simulink model "dynamicANN"  (R2019b)
settings: Solver=VariableStepAuto  StartTime=0.0  StopTime=3  RelTol=1e-3
values from neighbouring files (symbols this model uses):
  a = 87.548e-3    (= 0.087548)    [main.m]
  b = 132.452e-3    (= 0.132452)    [main.m]
  d = 22.452e-3    (= 0.022452)    [main.m]
  delta = 4e-6    (= 4e-06)    [main.m]
  F1 = mass*g-F2    (= 23.4474357109)    [main.m]
  F2 = a*mass*g/(a+b)    (= 15.4982642891)    [main.m]
  g = 9.81    [main.m]
  h0 = 75e-6    (= 7.5e-05)    [main.m]
  Jd = 0.047331604    [main.m]
  Jp = 0.00075    [main.m]
  Kps = (Vmax-Vmin)/(Hmax-Hmin)    (= 1666.66666667)    [main.m]
  Ksv = 30    [main.m]
  mass = 3.970    (= 3.97)    [main.m]
  mm = F2/g    (= 1.57984345455)    [main.m]
  omega = n_rpm*2*pi/60    (= 293.215314335)    [main.m]
  s = 30e-3    (= 0.03)    [main.m]
  tau = 0.12    [main.m]
  taus = 0.00125    [main.m]
  Ts = 1/fs    (= 0.001)    [main.m]
libraries: neural x480, simulink x2
(part 1 of 11)
settings Model: Creator=Alexander  LastModifiedBy=Alexander

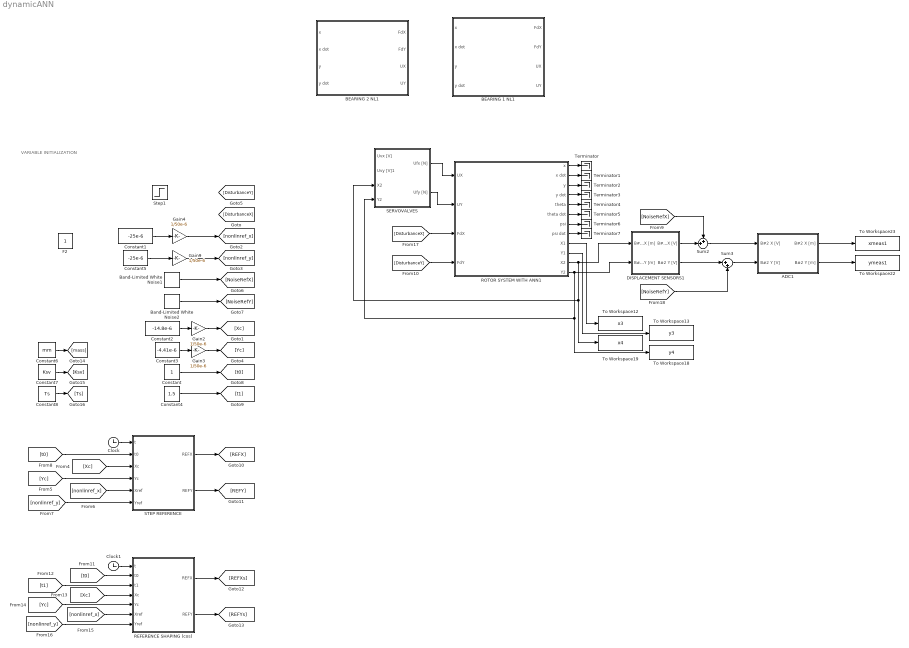
== system dynamicANN ==
  note: VARIABLE INITIALIZATION
  ADC1 : Subsystem
  BEARING 1 NL1 : Subsystem
  BEARING 2 NL1 : Subsystem
  Band-Limited White Noise1 : simulink/Sources/Band-Limited White Noise  Cov=n_pow  Ts=Ts  seed=[23341]
  Band-Limited White Noise2 : simulink/Sources/Band-Limited White Noise  Cov=n_pow  Ts=1.1*Ts  seed=[23341]
  Clock : Clock
  Clock1 : Clock
  Constant : Constant
  Constant1 : Constant  Value=-25e-6
  Constant2 : Constant  Value=-14.8e-6
  Constant3 : Constant  Value=-4.41e-6
  Constant4 : Constant  Value=1.5
  Constant5 : Constant  Value=-25e-6
  Constant6 : Constant  Value=mm
  Constant7 : Constant  Value=Ksv
  Constant8 : Constant  Value=Ts
  DISPLACEMENT SENSORS1 : Subsystem
  Gain{2..4,9} (4 alike) : Gain  Gain=1/50e-6
  REFERENCE SHAPING (cos) : MATLAB Function  TreatAsAtomicUnit=on
  ROTOR SYSTEM WITH ANN1 : Subsystem
  SERVOVALVES : Subsystem
  STEP REFERENCE : MATLAB Function  TreatAsAtomicUnit=on
  Step1 : Step  After=-10  SampleTime=0
  Sum2 : Sum  Inputs=++|
  Sum3 : Sum  Inputs=|++
  Terminator{,1..7} (8 alike) : Terminator
  To Workspace12 : ToWorkspace  VariableName=x3  SampleTime=-1
      settings: Save2DSignal=2-D array (concatenate along first dimension)
  To Workspace13 : ToWorkspace  VariableName=y3  SampleTime=-1
      settings: Save2DSignal=2-D array (concatenate along first dimension)
  To Workspace18 : ToWorkspace  VariableName=y4  SampleTime=-1
      settings: Save2DSignal=2-D array (concatenate along first dimension)
  To Workspace19 : ToWorkspace  VariableName=x4  SampleTime=-1
      settings: Save2DSignal=2-D array (concatenate along first dimension)
  To Workspace22 : ToWorkspace  VariableName=ymeas1  SampleTime=-1
      settings: Save2DSignal=2-D array (concatenate along first dimension)
  To Workspace23 : ToWorkspace  VariableName=xmeas1  SampleTime=-1
      settings: Save2DSignal=2-D array (concatenate along first dimension)
  F2 : Constant  IOType=siggen
  wires:
  Constant/1 -> [t0]
  Gain3/1 -> [Yc]
  Band-Limited White Noise2/1 -> [NoiseRefY]
  Band-Limited White Noise1/1 -> [NoiseRefX]
  Gain2/1 -> [Xc]
  [nonlinref_y] -> REFERENCE SHAPING (cos)/7(Yref)
  STEP REFERENCE/2(REFY) -> [REFY]
  Constant1/1 -> Gain4/1
  [Xc] -> REFERENCE SHAPING (cos)/4(Xc)
  [Yc] -> STEP REFERENCE/4(Yc)
  STEP REFERENCE/1(REFX) -> [REFX]
  Constant5/1 -> Gain9/1
  Gain9/1 -> [nonlinref_y]
  [nonlinref_y] -> STEP REFERENCE/6(Yref)
  Gain4/1 -> [nonlinref_x]
  REFERENCE SHAPING (cos)/2(REFY) -> [REFYs]
  [t1] -> REFERENCE SHAPING (cos)/3(t1)
  [Xc] -> STEP REFERENCE/3(Xc)
  [t0] -> REFERENCE SHAPING (cos)/2(t0)
  [t0] -> STEP REFERENCE/2(t0)
  [Yc] -> REFERENCE SHAPING (cos)/5(Yc)
  Constant6/1 -> [mass]
  [nonlinref_x] -> REFERENCE SHAPING (cos)/6(Xref)
  [nonlinref_x] -> STEP REFERENCE/5(Xref)
  Constant2/1 -> Gain2/1
  Constant3/1 -> Gain3/1
  Constant4/1 -> [t1]
  Clock/1 -> STEP REFERENCE/1(t)
  Constant8/1 -> [Ts]
  REFERENCE SHAPING (cos)/1(REFX) -> [REFXs]
  Constant7/1 -> [Ksv]
  Clock1/1 -> REFERENCE SHAPING (cos)/1(t)
  ROTOR SYSTEM WITH ANN1/11("X2 ") -> To Workspace19/1, SERVOVALVES/3(X2), DISPLACEMENT SENSORS1/1(B#2 X [m])
  SERVOVALVES/1(Ufx [N]) -> ROTOR SYSTEM WITH ANN1/1(UX)
  [DisturbanceX] -> ROTOR SYSTEM WITH ANN1/3(FdX)
  DISPLACEMENT SENSORS1/2(B#2 Y [V]) -> Sum3/1
  ROTOR SYSTEM WITH ANN1/12(Y2) -> SERVOVALVES/4(Y2), To Workspace18/1, DISPLACEMENT SENSORS1/2(B#2 Y [m])
  [NoiseRefY] -> Sum3/2
  DISPLACEMENT SENSORS1/1(B#2 X [V]) -> Sum2/2
  SERVOVALVES/2(Ufy [N]) -> ROTOR SYSTEM WITH ANN1/2(UY)
  Sum2/1 -> ADC1/1(B#2 X [V])
  ROTOR SYSTEM WITH ANN1/9(X1) -> To Workspace12/1
  ADC1/2(B#2 Y [m]) -> To Workspace22/1
  Sum3/1 -> ADC1/2(B#2 Y [V])
  [NoiseRefX] -> Sum2/1
  ROTOR SYSTEM WITH ANN1/10(Y1) -> To Workspace13/1
  [DisturbanceY] -> ROTOR SYSTEM WITH ANN1/4(FdY)
  ADC1/1(B#2 X [m]) -> To Workspace23/1
  ROTOR SYSTEM WITH ANN1/1("x ") -> Terminator/1
  ROTOR SYSTEM WITH ANN1/2(x dot) -> Terminator1/1
  ROTOR SYSTEM WITH ANN1/3(y) -> Terminator2/1
  ROTOR SYSTEM WITH ANN1/4(y dot) -> Terminator3/1
  ROTOR SYSTEM WITH ANN1/5(theta) -> Terminator4/1
  ROTOR SYSTEM WITH ANN1/6("theta dot ") -> Terminator5/1
  ROTOR SYSTEM WITH ANN1/7(psi) -> Terminator6/1
  ROTOR SYSTEM WITH ANN1/8(psi dot) -> Terminator7/1

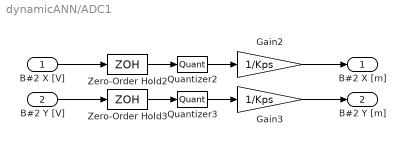
== system dynamicANN/ADC1 ==
  B#2 X [V] : Inport
  B#2 Y [V] : Inport  Port=2
  Gain2 : Gain  Gain=1/Kps
  Gain3 : Gain  Gain=1/Kps
  Quantizer2 : Quantizer  QuantizationInterval=0.000152587890625
  Quantizer3 : Quantizer  QuantizationInterval=0.000152587890625
  Zero-Order Hold2 : ZeroOrderHold  SampleTime=Ts
  Zero-Order Hold3 : ZeroOrderHold  SampleTime=Ts
  B#2 X [m] : Outport
  B#2 Y [m] : Outport  Port=2
  wires:
  Quantizer2/1 -> Gain2/1
  Quantizer3/1 -> Gain3/1
  B#2 X [V]/1 -> Zero-Order Hold2/1
  Gain2/1 -> B#2 X [m]/1
  Zero-Order Hold2/1 -> Quantizer2/1
  Gain3/1 -> B#2 Y [m]/1
  Zero-Order Hold3/1 -> Quantizer3/1
  B#2 Y [V]/1 -> Zero-Order Hold3/1

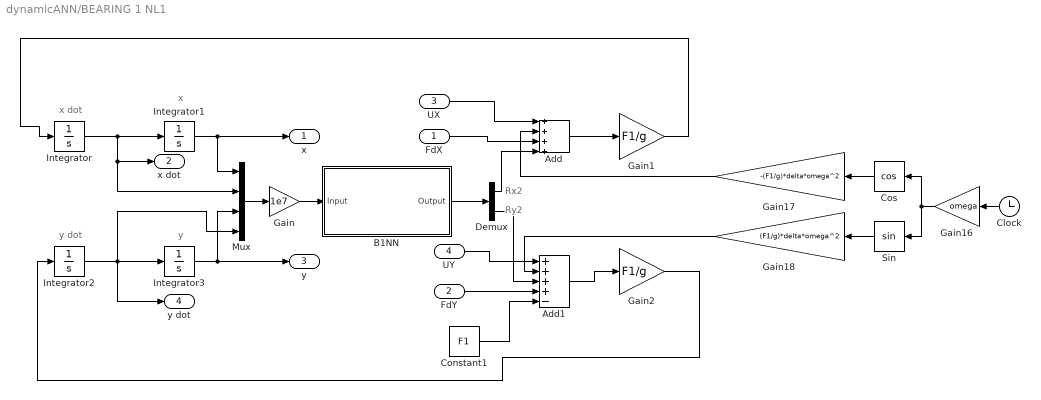
== system dynamicANN/BEARING 1 NL1 ==
  note: y
  note: x dot
  note: y dot
  note: Rx2
  note: Ry2
  note: x
  FdX : Inport
  FdY : Inport  Port=2
  UX : Inport  Port=3
  UY : Inport  Port=4
  Add : Sum  Inputs=++++
  Add1 : Sum  Inputs=++++-
  B1NN : Subsystem
      mask help: Feed-Forward Neural Network
      mask Display: e = 0.06;c1 = [120 150 230]/255;c2 = ([120 150 230]+0)/383;c3 = ([120 150 230]+128)/383;patch([0 1 1 0],[0 0 1 1],c1);patch([0 1 1 1-e 1-e 0+e],[0 0 1 1-e 0+e 0+e],c2);patch([0 0 1 1-e 0+e 0+e],[0 1 1 1-e 1-e 0+e],c3);plot([0 1 1 0 0],[0 0 1 1 0]);fprintf('B1 NNET');port_label('input',1,' X');port_label('output',1,'F ');
  Clock : Clock
  Constant1 : Constant  Value=F1
  Cos : Trigonometry  Operator=cos
  Demux : Demux  Outputs=2
  Gain : Gain  Gain=1e7
  Gain1 : Gain  Gain=F1/g
  Gain16 : Gain  Gain=omega
  Gain17 : Gain  Gain=-(F1/g)*delta*omega^2
  Gain18 : Gain  Gain=(F1/g)*delta*omega^2
  Gain2 : Gain  Gain=F1/g
  Integrator{,1..3} (4 alike) : Integrator
  Mux : Mux
  Sin : Trigonometry
  x : Outport
  "x dot " : Outport  Port=2
  y : Outport  Port=3
  y dot : Outport  Port=4
  wires:
  Mux/1 -> Gain/1
  B1NN/1(Output) -> Demux/1
  Gain/1 -> B1NN/1(Input)
  Integrator1/1 -> x/1, Mux/1
  Integrator2/1 -> y dot/1, Mux/4, Integrator3/1
  Integrator/1 -> "x dot "/1, Mux/2, Integrator1/1
  Integrator3/1 -> y/1, Mux/3
  Clock/1 -> Gain16/1
  Sin/1 -> Gain18/1
  Cos/1 -> Gain17/1
  Gain2/1 -> Integrator2/1
  Add/1 -> Gain1/1
  Gain16/1 -> Sin/1, Cos/1
  Add1/1 -> Gain2/1
  Gain17/1 -> Add/2
  Gain18/1 -> Add1/2
  Gain1/1 -> Integrator/1
  FdX/1 -> Add/3
  Demux/1 -> Add/4
  FdY/1 -> Add1/4
  Constant1/1 -> Add1/5
  UX/1 -> Add/1
  Demux/2 -> Add1/3
  UY/1 -> Add1/1

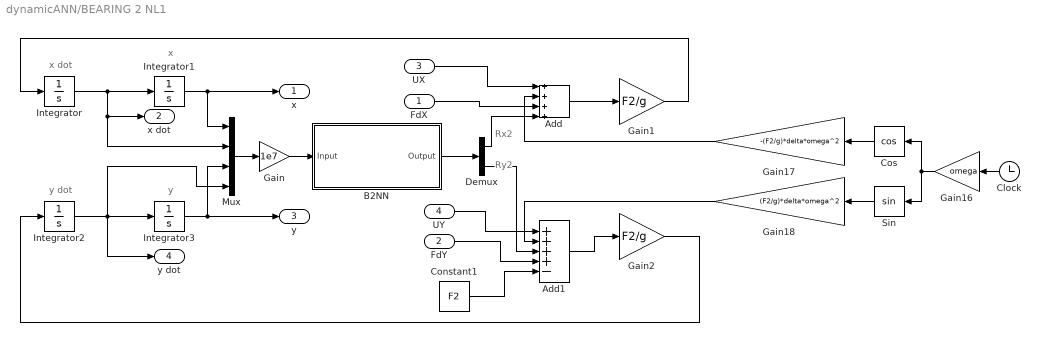
== system dynamicANN/BEARING 2 NL1 ==
  note: x
  note: x dot
  note: y
  note: y dot
  note: Ry2
  note: Rx2
  FdX : Inport
  FdY : Inport  Port=2
  UX : Inport  Port=3
  UY : Inport  Port=4
  Add : Sum  Inputs=++++
  Add1 : Sum  Inputs=++++-
  "B2NN " : Subsystem
      mask help: Feed-Forward Neural Network
      mask Display: e = 0.06;c1 = [120 150 230]/255;c2 = ([120 150 230]+0)/383;c3 = ([120 150 230]+128)/383;patch([0 1 1 0],[0 0 1 1],c1);patch([0 1 1 1-e 1-e 0+e],[0 0 1 1-e 0+e 0+e],c2);patch([0 0 1 1-e 0+e 0+e],[0 1 1 1-e 1-e 0+e],c3);plot([0 1 1 0 0],[0 0 1 1 0]);fprintf('B2 NNET');port_label('input',1,' X');port_label('output',1,'F ');
  Clock : Clock
  Constant1 : Constant  Value=F2
  Cos : Trigonometry  Operator=cos
  Demux : Demux  Outputs=2
  Gain : Gain  Gain=1e7
  Gain1 : Gain  Gain=F2/g
  Gain16 : Gain  Gain=omega
  Gain17 : Gain  Gain=-(F2/g)*delta*omega^2
  Gain18 : Gain  Gain=(F2/g)*delta*omega^2
  Gain2 : Gain  Gain=F2/g
  Integrator{,1..3} (4 alike) : Integrator
  Mux : Mux
  Sin : Trigonometry
  x : Outport
  "x dot " : Outport  Port=2
  y : Outport  Port=3
  y dot : Outport  Port=4
  wires:
  Add1/1 -> Gain2/1
  Gain1/1 -> Integrator/1
  FdY/1 -> Add1/4
  Integrator/1 -> "x dot "/1, Mux/2, Integrator1/1
  Integrator1/1 -> x/1, Mux/1
  Integrator2/1 -> y dot/1, Mux/4, Integrator3/1
  Add/1 -> Gain1/1
  Integrator3/1 -> y/1, Mux/3
  FdX/1 -> Add/3
  Mux/1 -> Gain/1
  Demux/2 -> Add1/3
  Gain/1 -> "B2NN "/1(Input)
  Demux/1 -> Add/4
  Gain2/1 -> Integrator2/1
  Constant1/1 -> Add1/5
  "B2NN "/1(Output) -> Demux/1
  Sin/1 -> Gain18/1
  Cos/1 -> Gain17/1
  Gain16/1 -> Sin/1, Cos/1
  Clock/1 -> Gain16/1
  Gain17/1 -> Add/2
  Gain18/1 -> Add1/2
  UX/1 -> Add/1
  UY/1 -> Add1/1

== system dynamicANN/DISPLACEMENT SENSORS1 ==
  B#2 X [m] : Inport
  B#2 Y [m] : Inport  Port=2
  Transfer Fcn2 : TransferFcn  Numerator=[Kps]  Denominator=[taus 1]
  Transfer Fcn3 : TransferFcn  Numerator=[Kps]  Denominator=[taus 1]
  B#2 X [V] : Outport
  B#2 Y [V] : Outport  Port=2
  wires:
  B#2 Y [m]/1 -> Transfer Fcn3/1
  B#2 X [m]/1 -> Transfer Fcn2/1
  Transfer Fcn2/1 -> B#2 X [V]/1
  Transfer Fcn3/1 -> B#2 Y [V]/1

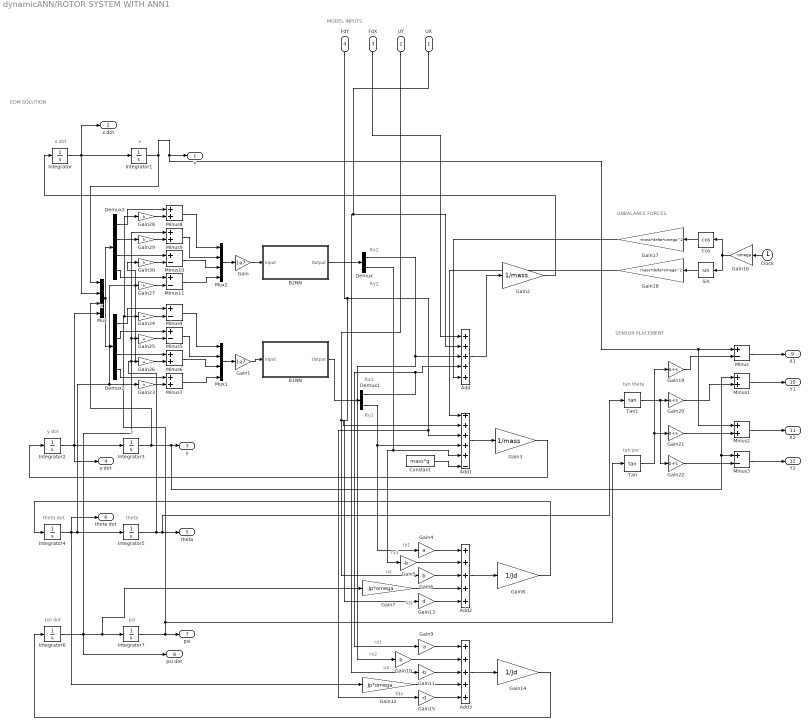
== system dynamicANN/ROTOR SYSTEM WITH ANN1 ==
  note: SENSOR PLACEMENT
  note: tan theta
  note: EOM SOLUTION
  note: MODEL INPUTS
  note: UNBALANCE FORCES
  note: fdx
  note: ux
  note: rx2
  note: rx1
  note: fdy
  note: uy
  note: ry2
  note: ry1
  note: Ry2
  note: Rx2
  note: X
  note: x dot
  note: x
  note: y
  note: y dot
  note: Ry1
  note: Rx1
  note: theta dot
  note: theta
  note: psi dot
  note: psi
  note: tan psi
  UX : Inport
  UY : Inport  Port=2
  FdX : Inport  Port=3
  FdY : Inport  Port=4
  Add : Sum  Inputs=+++++
  Add1 : Sum  Inputs=+++++-
  Add2 : Sum  Inputs=+++++
  Add3 : Sum  Inputs=+++++
  B1NN : Subsystem
      mask help: Feed-Forward Neural Network
      mask Display: e = 0.06;c1 = [120 150 230]/255;c2 = ([120 150 230]+0)/383;c3 = ([120 150 230]+128)/383;patch([0 1 1 0],[0 0 1 1],c1);patch([0 1 1 1-e 1-e 0+e],[0 0 1 1-e 0+e 0+e],c2);patch([0 0 1 1-e 0+e 0+e],[0 1 1 1-e 1-e 0+e],c3);plot([0 1 1 0 0],[0 0 1 1 0]);fprintf('B1 NNET');port_label('input',1,' X');port_label('output',1,'F ');
  "B2NN " : Subsystem
      mask help: Feed-Forward Neural Network
      mask Display: e = 0.06;c1 = [120 150 230]/255;c2 = ([120 150 230]+0)/383;c3 = ([120 150 230]+128)/383;patch([0 1 1 0],[0 0 1 1],c1);patch([0 1 1 1-e 1-e 0+e],[0 0 1 1-e 0+e 0+e],c2);patch([0 0 1 1-e 0+e 0+e],[0 1 1 1-e 1-e 0+e],c3);plot([0 1 1 0 0],[0 0 1 1 0]);fprintf('B2 NNET');port_label('input',1,' X');port_label('output',1,'F ');
  Clock : Clock
  Constant : Constant  Value=mass*g
  Cos : Trigonometry  Operator=cos
  Demux : Demux  Outputs=2
  Demux1 : Demux  Outputs=2
  Demux2 : Demux
  Demux3 : Demux
  Gain : Gain  Gain=1e7
  Gain1 : Gain  Gain=1e7
  Gain{6,10,27..30} (6 alike) : Gain  Gain=b
  Gain11 : Gain  Gain=-b
  Gain12 : Gain  Gain=Jp*omega
  Gain13 : Gain  Gain=d
  Gain14 : Gain  Gain=1/Jd
  Gain15 : Gain  Gain=-d
  Gain16 : Gain  Gain=omega
  Gain17 : Gain  Gain=-mass*delta*omega^2
  Gain18 : Gain  Gain=mass*delta*omega^2
  Gain19 : Gain  Gain=a+s
  Gain2 : Gain  Gain=1/mass
  Gain20 : Gain  Gain=a+s
  Gain21 : Gain  Gain=b+s
  Gain22 : Gain  Gain=b+s
  Gain{4,23..26} (5 alike) : Gain  Gain=a
  Gain3 : Gain  Gain=1/mass
  Gain5 : Gain  Gain=-b
  Gain7 : Gain  Gain=-Jp*omega
  Gain8 : Gain  Gain=1/Jd
  Gain9 : Gain  Gain=-a
  Integrator{,1..7} (8 alike) : Integrator
  Minus{,3..5,10..11} (6 alike) : Sum  Inputs=+-
  Minus{1..2,6..9} (6 alike) : Sum
  Mux : Mux
  Mux1 : Mux
  Mux2 : Mux
  Sin : Trigonometry
  Tan : Trigonometry  Operator=tan
  Tan1 : Trigonometry  Operator=tan
  "x " : Outport
  x dot : Outport  Port=2
  y : Outport  Port=3
  y dot : Outport  Port=4
  theta : Outport  Port=5
  "theta dot " : Outport  Port=6
  psi : Outport  Port=7
  psi dot : Outport  Port=8
  X1 : Outport  Port=9
  Y1 : Outport  Port=10
  "X2 " : Outport  Port=11
  Y2 : Outport  Port=12
  wires:
  FdY/1 -> Gain15/1, Add1/3, Gain13/1
  Integrator2/1 -> Mux/4, y dot/1, Integrator3/1
  Integrator3/1 -> Minus1/1, Minus3/1, y/1, Mux/3
  Integrator4/1 -> Gain23/1, Gain27/1, Integrator5/1, Gain12/1, "theta dot "/1
  Integrator6/1 -> psi dot/1, Gain7/1, Integrator7/1, Gain29/1, Gain25/1
  Mux/1 -> Demux2/1, Demux3/1
  Add3/1 -> Gain14/1
  UX/1 -> Gain11/1, Add/2
  Add/1 -> Gain2/1
  Demux1/2 -> Gain4/1, Add1/4
  Gain15/1 -> Add3/5
  Integrator/1 -> x dot/1, Mux/2, Integrator1/1
  Demux/1 -> Gain10/1, Add/3
  UY/1 -> Add1/2, Gain6/1
  Integrator7/1 -> Gain24/1, Gain28/1, Tan/1, psi/1
  Gain/1 -> "B2NN "/1(Input)
  Gain11/1 -> Add3/3
  Gain12/1 -> Add3/4
  Gain6/1 -> Add2/3
  Gain10/1 -> Add3/2
  Gain9/1 -> Add3/1
  Demux/2 -> Gain5/1, Add1/5
  Add1/1 -> Gain3/1
  B1NN/1(Output) -> Demux1/1
  Gain8/1 -> Integrator4/1
  Integrator1/1 -> "x "/1, Minus2/1, Minus/1, Mux/1
  FdX/1 -> Add/1
  Demux1/1 -> Gain9/1, Add/4
  Add2/1 -> Gain8/1
  "B2NN "/1(Output) -> Demux/1
  Gain13/1 -> Add2/5
  Gain1/1 -> B1NN/1(Input)
  Gain3/1 -> Integrator2/1
  Gain4/1 -> Add2/1
  Gain7/1 -> Add2/4
  Gain5/1 -> Add2/2
  Gain14/1 -> Integrator6/1
  Gain2/1 -> Integrator/1
  Integrator5/1 -> Gain30/1, Gain26/1, Tan1/1, theta/1
  Constant/1 -> Add1/6
  Clock/1 -> Gain16/1
  Gain16/1 -> Sin/1, Cos/1
  Cos/1 -> Gain17/1
  Sin/1 -> Gain18/1
  Gain17/1 -> Add/5
  Gain18/1 -> Add1/1
  Gain19/1 -> Minus/2
  Tan/1 -> Gain19/1, Gain21/1
  Minus/1 -> X1/1
  Tan1/1 -> Gain22/1, Gain20/1
  Gain20/1 -> Minus1/2
  Minus1/1 -> Y1/1
  Gain21/1 -> Minus2/2
  Minus2/1 -> "X2 "/1
  Minus3/1 -> Y2/1
  Gain22/1 -> Minus3/2
  Mux1/1 -> Gain1/1
  Minus4/1 -> Mux1/1
  Minus5/1 -> Mux1/2
  Minus7/1 -> Mux1/4
  Minus6/1 -> Mux1/3
  Gain24/1 -> Minus4/2
  Gain25/1 -> Minus5/2
  Gain23/1 -> Minus7/2
  Demux2/1 -> Minus4/1
  Demux2/2 -> Minus5/1
  Demux2/3 -> Minus6/1
  Gain26/1 -> Minus6/2
  Demux2/4 -> Minus7/1
  Gain29/1 -> Minus9/2
  Gain28/1 -> Minus8/2
  Minus8/1 -> Mux2/1
  Gain30/1 -> Minus10/2
  Demux3/3 -> Minus10/1
  Minus10/1 -> Mux2/3
  Demux3/2 -> Minus9/1
  Demux3/4 -> Minus11/1
  Demux3/1 -> Minus8/1
  Minus9/1 -> Mux2/2
  Gain27/1 -> Minus11/2
  Mux2/1 -> Gain/1
  Minus11/1 -> Mux2/4

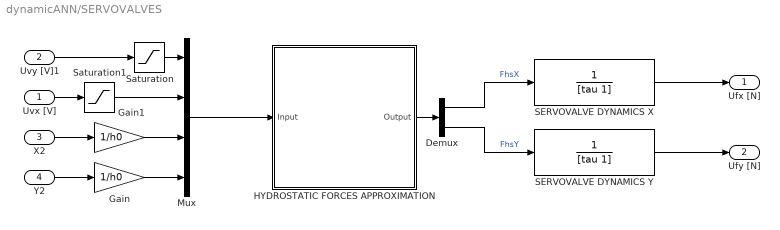
== system dynamicANN/SERVOVALVES ==
  Uvx [V] : Inport
  Uvy [V]1 : Inport  Port=2
  X2 : Inport  Port=3
  Y2 : Inport  Port=4
  Demux : Demux  Outputs=2
  Gain : Gain  Gain=1/h0
  Gain1 : Gain  Gain=1/h0
  HYDROSTATIC FORCES APPROXIMATION : Subsystem
      mask help: Function Fitting Neural Network
      mask Display: e = 0.06;c1 = [120 150 230]/255;c2 = ([120 150 230]+0)/383;c3 = ([120 150 230]+128)/383;patch([0 1 1 0],[0 0 1 1],c1);patch([0 1 1 1-e 1-e 0+e],[0 0 1 1-e 0+e 0+e],c2);patch([0 0 1 1-e 0+e 0+e],[0 1 1 1-e 1-e 0+e],c3);plot([0 1 1 0 0],[0 0 1 1 0]);fprintf('NNET');port_label('input',1,' Input');port_label('output',1,'Output ');
  Mux : Mux
  SERVOVALVE DYNAMICS X : TransferFcn  Numerator=1  Denominator=[tau 1]
  SERVOVALVE DYNAMICS Y : TransferFcn  Numerator=1  Denominator=[tau 1]
  Saturation : Saturate  UpperLimit=10  LowerLimit=0
  Saturation1 : Saturate  UpperLimit=10  LowerLimit=0
  Ufx [N] : Outport
  Ufy [N] : Outport  Port=2
  wires:
  SERVOVALVE DYNAMICS X/1 -> Ufx [N]/1
  HYDROSTATIC FORCES APPROXIMATION/1(Output) -> Demux/1
  Demux/1 -> SERVOVALVE DYNAMICS X/1  "FhsX"
  Demux/2 -> SERVOVALVE DYNAMICS Y/1  "FhsY"
  SERVOVALVE DYNAMICS Y/1 -> Ufy [N]/1
  Mux/1 -> HYDROSTATIC FORCES APPROXIMATION/1(Input)
  Y2/1 -> Gain/1
  X2/1 -> Gain1/1
  Uvx [V]/1 -> Saturation1/1
  Uvy [V]1/1 -> Saturation/1
  Gain/1 -> Mux/4
  Gain1/1 -> Mux/3
  Saturation/1 -> Mux/1
  Saturation1/1 -> Mux/2

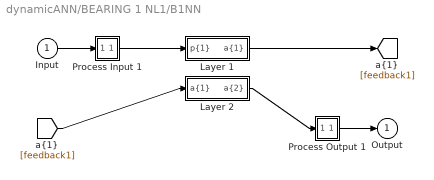
== system dynamicANN/BEARING 1 NL1/B1NN ==
  Input : Inport  PortDimensions=4
      mask Display: e = 0.06;c1 = [120 230 180]/255;c2 = ([120 230 180]+0)/(256+128);c3 = ([120 230 180]+128)/(256+128);patch([0 1 1 0],[0 0 1 1],c1);patch([0 1 1 1-e 1-e 0+e],[0 0 1 1-e 0+e 0+e],c2);patch([0 0 1 1-e 0+e 0+e],[0 1 1 1-e 1-e 0+e],c3);plot([0 1 1 0 0],[0 0 1 1 0]);
  Layer 1 : Subsystem
      mask Display: e = 0.06;c1 = [120 150 230]/255;c2 = ([120 150 230]+0)/383;c3 = ([120 150 230]+128)/383;patch([0 1 1 0],[0 0 1 1],c1);patch([0 1 1 1-e 1-e 0+e],[0 0 1 1-e 0+e 0+e],c2);patch([0 0 1 1-e 0+e 0+e],[0 1 1 1-e 1-e 0+e],c3);plot([0 1 1 0 0],[0 0 1 1 0]);
  Layer 2 : Subsystem
      mask Display: e = 0.06;c1 = [120 150 230]/255;c2 = ([120 150 230]+0)/383;c3 = ([120 150 230]+128)/383;patch([0 1 1 0],[0 0 1 1],c1);patch([0 1 1 1-e 1-e 0+e],[0 0 1 1-e 0+e 0+e],c2);patch([0 0 1 1-e 0+e 0+e],[0 1 1 1-e 1-e 0+e],c3);plot([0 1 1 0 0],[0 0 1 1 0]);
  Process Input 1 : Subsystem
      mask Display: e = 0.06;c1 = [120 150 230]/255;c2 = ([120 150 230]+0)/383;c3 = ([120 150 230]+128)/383;patch([0 1 1 0],[0 0 1 1],c1);patch([0 1 1 1-e 1-e 0+e],[0 0 1 1-e 0+e 0+e],c2);patch([0 0 1 1-e 0+e 0+e],[0 1 1 1-e 1-e 0+e],c3);plot([0 1 1 0 0],[0 0 1 1 0]);
  Process Output 1 : Subsystem
      mask Display: e = 0.06;c1 = [120 150 230]/255;c2 = ([120 150 230]+0)/383;c3 = ([120 150 230]+128)/383;patch([0 1 1 0],[0 0 1 1],c1);patch([0 1 1 1-e 1-e 0+e],[0 0 1 1-e 0+e 0+e],c2);patch([0 0 1 1-e 0+e 0+e],[0 1 1 1-e 1-e 0+e],c3);plot([0 1 1 0 0],[0 0 1 1 0]);
  Output : Outport  InitialOutput=[0;0]
      mask Display: e = 0.06;c1 = [120 230 180]/255;c2 = ([120 230 180]+0)/(256+128);c3 = ([120 230 180]+128)/(256+128);patch([0 1 1 0],[0 0 1 1],c1);patch([0 1 1 1-e 1-e 0+e],[0 0 1 1-e 0+e 0+e],c2);patch([0 0 1 1-e 0+e 0+e],[0 1 1 1-e 1-e 0+e],c3);plot([0 1 1 0 0],[0 0 1 1 0]);
  wires:
  Input/1 -> Process Input 1/1(x)
  Process Output 1/1(y) -> Output/1
  Process Input 1/1(p) -> Layer 1/1("p{1}")
  Layer 1/1("a{1}") -> [feedback1]
  [feedback1] -> Layer 2/1("a{1} ")
  Layer 2/1("a{2}") -> Process Output 1/1(a)

== system dynamicANN/BEARING 2 NL1/B2NN  ==
  Input : Inport  PortDimensions=4
      mask Display: e = 0.06;c1 = [120 230 180]/255;c2 = ([120 230 180]+0)/(256+128);c3 = ([120 230 180]+128)/(256+128);patch([0 1 1 0],[0 0 1 1],c1);patch([0 1 1 1-e 1-e 0+e],[0 0 1 1-e 0+e 0+e],c2);patch([0 0 1 1-e 0+e 0+e],[0 1 1 1-e 1-e 0+e],c3);plot([0 1 1 0 0],[0 0 1 1 0]);
  Layer 1 : Subsystem
      mask Display: e = 0.06;c1 = [120 150 230]/255;c2 = ([120 150 230]+0)/383;c3 = ([120 150 230]+128)/383;patch([0 1 1 0],[0 0 1 1],c1);patch([0 1 1 1-e 1-e 0+e],[0 0 1 1-e 0+e 0+e],c2);patch([0 0 1 1-e 0+e 0+e],[0 1 1 1-e 1-e 0+e],c3);plot([0 1 1 0 0],[0 0 1 1 0]);
  Layer 2 : Subsystem
      mask Display: e = 0.06;c1 = [120 150 230]/255;c2 = ([120 150 230]+0)/383;c3 = ([120 150 230]+128)/383;patch([0 1 1 0],[0 0 1 1],c1);patch([0 1 1 1-e 1-e 0+e],[0 0 1 1-e 0+e 0+e],c2);patch([0 0 1 1-e 0+e 0+e],[0 1 1 1-e 1-e 0+e],c3);plot([0 1 1 0 0],[0 0 1 1 0]);
  Process Input 1 : Subsystem
      mask Display: e = 0.06;c1 = [120 150 230]/255;c2 = ([120 150 230]+0)/383;c3 = ([120 150 230]+128)/383;patch([0 1 1 0],[0 0 1 1],c1);patch([0 1 1 1-e 1-e 0+e],[0 0 1 1-e 0+e 0+e],c2);patch([0 0 1 1-e 0+e 0+e],[0 1 1 1-e 1-e 0+e],c3);plot([0 1 1 0 0],[0 0 1 1 0]);
  Process Output 1 : Subsystem
      mask Display: e = 0.06;c1 = [120 150 230]/255;c2 = ([120 150 230]+0)/383;c3 = ([120 150 230]+128)/383;patch([0 1 1 0],[0 0 1 1],c1);patch([0 1 1 1-e 1-e 0+e],[0 0 1 1-e 0+e 0+e],c2);patch([0 0 1 1-e 0+e 0+e],[0 1 1 1-e 1-e 0+e],c3);plot([0 1 1 0 0],[0 0 1 1 0]);
  Output : Outport  InitialOutput=[0;0]
      mask Display: e = 0.06;c1 = [120 230 180]/255;c2 = ([120 230 180]+0)/(256+128);c3 = ([120 230 180]+128)/(256+128);patch([0 1 1 0],[0 0 1 1],c1);patch([0 1 1 1-e 1-e 0+e],[0 0 1 1-e 0+e 0+e],c2);patch([0 0 1 1-e 0+e 0+e],[0 1 1 1-e 1-e 0+e],c3);plot([0 1 1 0 0],[0 0 1 1 0]);
  wires:
  Input/1 -> Process Input 1/1(x)
  Process Output 1/1(y) -> Output/1
  Process Input 1/1(p) -> Layer 1/1("p{1}")
  Layer 1/1("a{1}") -> [feedback1]
  [feedback1] -> Layer 2/1("a{1} ")
  Layer 2/1("a{2}") -> Process Output 1/1(a)

== system dynamicANN/ROTOR SYSTEM WITH ANN1/B1NN ==
  Input : Inport  PortDimensions=4
      mask Display: e = 0.06;c1 = [120 230 180]/255;c2 = ([120 230 180]+0)/(256+128);c3 = ([120 230 180]+128)/(256+128);patch([0 1 1 0],[0 0 1 1],c1);patch([0 1 1 1-e 1-e 0+e],[0 0 1 1-e 0+e 0+e],c2);patch([0 0 1 1-e 0+e 0+e],[0 1 1 1-e 1-e 0+e],c3);plot([0 1 1 0 0],[0 0 1 1 0]);
  Layer 1 : Subsystem
      mask Display: e = 0.06;c1 = [120 150 230]/255;c2 = ([120 150 230]+0)/383;c3 = ([120 150 230]+128)/383;patch([0 1 1 0],[0 0 1 1],c1);patch([0 1 1 1-e 1-e 0+e],[0 0 1 1-e 0+e 0+e],c2);patch([0 0 1 1-e 0+e 0+e],[0 1 1 1-e 1-e 0+e],c3);plot([0 1 1 0 0],[0 0 1 1 0]);
  Layer 2 : Subsystem
      mask Display: e = 0.06;c1 = [120 150 230]/255;c2 = ([120 150 230]+0)/383;c3 = ([120 150 230]+128)/383;patch([0 1 1 0],[0 0 1 1],c1);patch([0 1 1 1-e 1-e 0+e],[0 0 1 1-e 0+e 0+e],c2);patch([0 0 1 1-e 0+e 0+e],[0 1 1 1-e 1-e 0+e],c3);plot([0 1 1 0 0],[0 0 1 1 0]);
  Process Input 1 : Subsystem
      mask Display: e = 0.06;c1 = [120 150 230]/255;c2 = ([120 150 230]+0)/383;c3 = ([120 150 230]+128)/383;patch([0 1 1 0],[0 0 1 1],c1);patch([0 1 1 1-e 1-e 0+e],[0 0 1 1-e 0+e 0+e],c2);patch([0 0 1 1-e 0+e 0+e],[0 1 1 1-e 1-e 0+e],c3);plot([0 1 1 0 0],[0 0 1 1 0]);
  Process Output 1 : Subsystem
      mask Display: e = 0.06;c1 = [120 150 230]/255;c2 = ([120 150 230]+0)/383;c3 = ([120 150 230]+128)/383;patch([0 1 1 0],[0 0 1 1],c1);patch([0 1 1 1-e 1-e 0+e],[0 0 1 1-e 0+e 0+e],c2);patch([0 0 1 1-e 0+e 0+e],[0 1 1 1-e 1-e 0+e],c3);plot([0 1 1 0 0],[0 0 1 1 0]);
  Output : Outport  InitialOutput=[0;0]
      mask Display: e = 0.06;c1 = [120 230 180]/255;c2 = ([120 230 180]+0)/(256+128);c3 = ([120 230 180]+128)/(256+128);patch([0 1 1 0],[0 0 1 1],c1);patch([0 1 1 1-e 1-e 0+e],[0 0 1 1-e 0+e 0+e],c2);patch([0 0 1 1-e 0+e 0+e],[0 1 1 1-e 1-e 0+e],c3);plot([0 1 1 0 0],[0 0 1 1 0]);
  wires:
  Input/1 -> Process Input 1/1(x)
  Process Output 1/1(y) -> Output/1
  Process Input 1/1(p) -> Layer 1/1("p{1}")
  Layer 1/1("a{1}") -> [feedback1]
  [feedback1] -> Layer 2/1("a{1} ")
  Layer 2/1("a{2}") -> Process Output 1/1(a)

== system dynamicANN/ROTOR SYSTEM WITH ANN1/B2NN  ==
  Input : Inport  PortDimensions=4
      mask Display: e = 0.06;c1 = [120 230 180]/255;c2 = ([120 230 180]+0)/(256+128);c3 = ([120 230 180]+128)/(256+128);patch([0 1 1 0],[0 0 1 1],c1);patch([0 1 1 1-e 1-e 0+e],[0 0 1 1-e 0+e 0+e],c2);patch([0 0 1 1-e 0+e 0+e],[0 1 1 1-e 1-e 0+e],c3);plot([0 1 1 0 0],[0 0 1 1 0]);
  Layer 1 : Subsystem
      mask Display: e = 0.06;c1 = [120 150 230]/255;c2 = ([120 150 230]+0)/383;c3 = ([120 150 230]+128)/383;patch([0 1 1 0],[0 0 1 1],c1);patch([0 1 1 1-e 1-e 0+e],[0 0 1 1-e 0+e 0+e],c2);patch([0 0 1 1-e 0+e 0+e],[0 1 1 1-e 1-e 0+e],c3);plot([0 1 1 0 0],[0 0 1 1 0]);
  Layer 2 : Subsystem
      mask Display: e = 0.06;c1 = [120 150 230]/255;c2 = ([120 150 230]+0)/383;c3 = ([120 150 230]+128)/383;patch([0 1 1 0],[0 0 1 1],c1);patch([0 1 1 1-e 1-e 0+e],[0 0 1 1-e 0+e 0+e],c2);patch([0 0 1 1-e 0+e 0+e],[0 1 1 1-e 1-e 0+e],c3);plot([0 1 1 0 0],[0 0 1 1 0]);
  Process Input 1 : Subsystem
      mask Display: e = 0.06;c1 = [120 150 230]/255;c2 = ([120 150 230]+0)/383;c3 = ([120 150 230]+128)/383;patch([0 1 1 0],[0 0 1 1],c1);patch([0 1 1 1-e 1-e 0+e],[0 0 1 1-e 0+e 0+e],c2);patch([0 0 1 1-e 0+e 0+e],[0 1 1 1-e 1-e 0+e],c3);plot([0 1 1 0 0],[0 0 1 1 0]);
  Process Output 1 : Subsystem
      mask Display: e = 0.06;c1 = [120 150 230]/255;c2 = ([120 150 230]+0)/383;c3 = ([120 150 230]+128)/383;patch([0 1 1 0],[0 0 1 1],c1);patch([0 1 1 1-e 1-e 0+e],[0 0 1 1-e 0+e 0+e],c2);patch([0 0 1 1-e 0+e 0+e],[0 1 1 1-e 1-e 0+e],c3);plot([0 1 1 0 0],[0 0 1 1 0]);
  Output : Outport  InitialOutput=[0;0]
      mask Display: e = 0.06;c1 = [120 230 180]/255;c2 = ([120 230 180]+0)/(256+128);c3 = ([120 230 180]+128)/(256+128);patch([0 1 1 0],[0 0 1 1],c1);patch([0 1 1 1-e 1-e 0+e],[0 0 1 1-e 0+e 0+e],c2);patch([0 0 1 1-e 0+e 0+e],[0 1 1 1-e 1-e 0+e],c3);plot([0 1 1 0 0],[0 0 1 1 0]);
  wires:
  Input/1 -> Process Input 1/1(x)
  Process Output 1/1(y) -> Output/1
  Process Input 1/1(p) -> Layer 1/1("p{1}")
  Layer 1/1("a{1}") -> [feedback1]
  [feedback1] -> Layer 2/1("a{1} ")
  Layer 2/1("a{2}") -> Process Output 1/1(a)

== system dynamicANN/SERVOVALVES/HYDROSTATIC FORCES APPROXIMATION ==
  Input : Inport  PortDimensions=4
      mask Display: e = 0.06;c1 = [120 230 180]/255;c2 = ([120 230 180]+0)/(256+128);c3 = ([120 230 180]+128)/(256+128);patch([0 1 1 0],[0 0 1 1],c1);patch([0 1 1 1-e 1-e 0+e],[0 0 1 1-e 0+e 0+e],c2);patch([0 0 1 1-e 0+e 0+e],[0 1 1 1-e 1-e 0+e],c3);plot([0 1 1 0 0],[0 0 1 1 0]);
  Layer 1 : Subsystem
      mask Display: e = 0.06;c1 = [120 150 230]/255;c2 = ([120 150 230]+0)/383;c3 = ([120 150 230]+128)/383;patch([0 1 1 0],[0 0 1 1],c1);patch([0 1 1 1-e 1-e 0+e],[0 0 1 1-e 0+e 0+e],c2);patch([0 0 1 1-e 0+e 0+e],[0 1 1 1-e 1-e 0+e],c3);plot([0 1 1 0 0],[0 0 1 1 0]);
  Layer 2 : Subsystem
      mask Display: e = 0.06;c1 = [120 150 230]/255;c2 = ([120 150 230]+0)/383;c3 = ([120 150 230]+128)/383;patch([0 1 1 0],[0 0 1 1],c1);patch([0 1 1 1-e 1-e 0+e],[0 0 1 1-e 0+e 0+e],c2);patch([0 0 1 1-e 0+e 0+e],[0 1 1 1-e 1-e 0+e],c3);plot([0 1 1 0 0],[0 0 1 1 0]);
  Process Input 1 : Subsystem
      mask Display: e = 0.06;c1 = [120 150 230]/255;c2 = ([120 150 230]+0)/383;c3 = ([120 150 230]+128)/383;patch([0 1 1 0],[0 0 1 1],c1);patch([0 1 1 1-e 1-e 0+e],[0 0 1 1-e 0+e 0+e],c2);patch([0 0 1 1-e 0+e 0+e],[0 1 1 1-e 1-e 0+e],c3);plot([0 1 1 0 0],[0 0 1 1 0]);
  Process Output 1 : Subsystem
      mask Display: e = 0.06;c1 = [120 150 230]/255;c2 = ([120 150 230]+0)/383;c3 = ([120 150 230]+128)/383;patch([0 1 1 0],[0 0 1 1],c1);patch([0 1 1 1-e 1-e 0+e],[0 0 1 1-e 0+e 0+e],c2);patch([0 0 1 1-e 0+e 0+e],[0 1 1 1-e 1-e 0+e],c3);plot([0 1 1 0 0],[0 0 1 1 0]);
  Output : Outport  InitialOutput=[0;0]
      mask Display: e = 0.06;c1 = [120 230 180]/255;c2 = ([120 230 180]+0)/(256+128);c3 = ([120 230 180]+128)/(256+128);patch([0 1 1 0],[0 0 1 1],c1);patch([0 1 1 1-e 1-e 0+e],[0 0 1 1-e 0+e 0+e],c2);patch([0 0 1 1-e 0+e 0+e],[0 1 1 1-e 1-e 0+e],c3);plot([0 1 1 0 0],[0 0 1 1 0]);
  wires:
  Input/1 -> Process Input 1/1(x)
  Process Output 1/1(y) -> Output/1
  Process Input 1/1(p) -> Layer 1/1("p{1}")
  Layer 1/1("a{1}") -> [feedback1]
  [feedback1] -> Layer 2/1("a{1} ")
  Layer 2/1("a{2}") -> Process Output 1/1(a)

== system dynamicANN/BEARING 1 NL1/B1NN/Layer 1 ==
  "p{1}" : Inport  PortDimensions=4
      mask Display: e = 0.06;c1 = [120 230 180]/255;c2 = ([120 230 180]+0)/(256+128);c3 = ([120 230 180]+128)/(256+128);patch([0 1 1 0],[0 0 1 1],c1);patch([0 1 1 1-e 1-e 0+e],[0 0 1 1-e 0+e 0+e],c2);patch([0 0 1 1-e 0+e 0+e],[0 1 1 1-e 1-e 0+e],c3);plot([0 1 1 0 0],[0 0 1 1 0]);
  Delays 1 : Subsystem
      mask Display: e = 0.06;c1 = [120 150 230]/255;c2 = ([120 150 230]+0)/383;c3 = ([120 150 230]+128)/383;patch([0 1 1 0],[0 0 1 1],c1);patch([0 1 1 1-e 1-e 0+e],[0 0 1 1-e 0+e 0+e],c2);patch([0 0 1 1-e 0+e 0+e],[0 1 1 1-e 1-e 0+e],c3);plot([0 1 1 0 0],[0 0 1 1 0]);disp('0');
  "IW{1,1}" : Subsystem
      mask Display: e = 0.06;c1 = [120 150 230]/255;c2 = ([120 150 230]+0)/383;c3 = ([120 150 230]+128)/383;patch([0 1 1 0],[0 0 1 1],c1);patch([0 1 1 1-e 1-e 0+e],[0 0 1 1-e 0+e 0+e],c2);patch([0 0 1 1-e 0+e 0+e],[0 1 1 1-e 1-e 0+e],c3);plot([0 1 1 0 0],[0 0 1 1 0]);disp('W');
  "b{1}" : Constant  Value=[-0.269837114600812888465242167512769810855388641357421875;1.1009012959734210124196351898717693984508514404296875;0.0166209802282058262401509551864364766515791416168212890625;0.28159769815177393414984408082091249525547027587890625;-0.243085988363765326258914001300581730902194976806640625;-0.472657677362091133144161858581355772912502288818359375;0.1799668095310359150484913470791070722043514251708984375;-0.77460523103353706719786941903294064104557037353515625;-0.048235427820019334543832911776917171664535999298095703125;0.59339758100700035203800553063047118484973907470703125;-0.155094531396554990987368682908709160983562469482421875;1.6006036137728061330420814556418918073177337646484375;1.7752998116072673528975656154216267168521881103515625;1.3037109320190960470853269725921563804149627685546875;0.8388055000069194466760791328852064907550811767578125;-0.302223958808178705393032714709988795220851898193359375;-0.45694166709408767790279171094880439341068267822265625;-4.2908799074421271058099591755308210849761962890625;-1.8004038624503182486336072543053887784481048583984375;-0.70518336433658179718264591429033316671848297119140625;0.298737623902642468465273850597441196441650390625;-2.55542627808326106020331280888058245182037353515625;0.1073398400688150566839595967394416220486164093017578125;-1.422179112793325206354211331927217543125152587890625;0.0310124388374934077672318011309471330605447292327880859375;0.9065679250558089652400894919992424547672271728515625;0.081681183749521102388513327241525985300540924072265625;-1.694355252055798732868652223260141909122467041015625;-1.4741584153405791202118280125432647764682769775390625;0.7012954069353292130273302973364479839801788330078125;0.12828256938603310732815998562728054821491241455078125;-0.94814500284482183811718414290226064622402191162109375;0.764940182751946196049175341613590717315673828125;2.367408736788062295630652442923747003078460693359375;-0.0141002096712693515689895917830654070712625980377197265625;1.2971081388031604486599235315225087106227874755859375;-3.2293610650964783559402349055744707584381103515625;-1.388359527561940698348053047084249556064605712890625;-1.336440475233187985537597342045046389102935791015625;3.49615742256232575613239532685838639736175537109375;-3.108220870068802543784158842754550278186798095703125;-2.77259867968769935231421186472289264202117919921875;0.313838660438552352616170537658035755157470703125;-0.2280135903292142829368316370164393447339534759521484375;-0.84307716841838387100693807951756753027439117431640625;0.11961594210892100009768768131834804080426692962646484375;2.325932793722724323259853917988948523998260498046875;1.547605345947079769075571675784885883331298828125;0.053231212578994983875002589002178865484893321990966796875;0.444768917748370518072675849907682277262210845947265625;0.491784220354247736395336687564849853515625;1.15691956493156578034131598542444407939910888671875;-0.9422832036139421330034338097902946174144744873046875;-0.538037449910673704067676226259209215641021728515625;1.4231843310200587016112194760353304445743560791015625;0.07763725068166793530366476261406205594539642333984375;1.637239552568078071459467537351883947849273681640625;0.10998363255999347998237425372280995361506938934326171875;2.032200702252918045331853136303834617137908935546875;-1.3039157691731950716729215855593793094158172607421875;0.98925726635870703251640634334762580692768096923828125;-2.067243191887783826388158558984287083148956298828125;0.254743809664128850744901910729822702705860137939453125;0.50517978684253861398900653512100689113140106201171875;1.51414754939552409496172913350164890289306640625;1.5288516227688864201894602956599555909633636474609375;-1.72494132371543340553898815414868295192718505859375;-2.42372811374729746347611580858938395977020263671875;6.24456533659202772668095349217765033245086669921875;0.363390884676975167710821779110119678080081939697265625;-3.377037389654569121688609811826609075069427490234375 ...(+1607 chars)]
      mask Display: e = 0.06;c1 = [120 150 230]/255;c2 = ([120 150 230]+0)/383;c3 = ([120 150 230]+128)/383;patch([0 1 1 0],[0 0 1 1],c1);patch([0 1 1 1-e 1-e 0+e],[0 0 1 1-e 0+e 0+e],c2);patch([0 0 1 1-e 0+e 0+e],[0 1 1 1-e 1-e 0+e],c3);plot([0 1 1 0 0],[0 0 1 1 0]);disp('b');
  netsum : Sum  Inputs=2  SaturateOnIntegerOverflow=on  InputSameDT=on  OutDataTypeStr=Inherit: Same as first input
      mask Display: e = 0.06;c1 = [120 150 230]/255;c2 = ([120 150 230]+0)/383;c3 = ([120 150 230]+128)/383;patch([0 1 1 0],[0 0 1 1],c1);patch([0 1 1 1-e 1-e 0+e],[0 0 1 1-e 0+e 0+e],c2);patch([0 0 1 1-e 0+e 0+e],[0 1 1 1-e 1-e 0+e],c3);plot([0 1 1 0 0],[0 0 1 1 0]);disp('+');
  tansig : neural/Transfer Functions/tansig
      settings: SourceProductName=Deep Learning Toolbox
  "a{1}" : Outport  InitialOutput=[0;0;0;0;0;0;0;0;0;0;0;0;0;0;0;0;0;0;0;0;0;0;0;0;0;0;0;0;0;0;0;0;0;0;0;0;0;0;0;0;0;0;0;0;0;0;0;0;0;0;0;0;0;0;0;0;0;0;0;0;0;0;0;0;0;0;0;0;0;0;0;0;0;0;0;0;0;0;0;0;0;0;0;0;0;0;0;0;0;0;0;0;0;0;0;0;0;0;0;0]
      mask Display: e = 0.06;c1 = [120 230 180]/255;c2 = ([120 230 180]+0)/(256+128);c3 = ([120 230 180]+128)/(256+128);patch([0 1 1 0],[0 0 1 1],c1);patch([0 1 1 1-e 1-e 0+e],[0 0 1 1-e 0+e 0+e],c2);patch([0 0 1 1-e 0+e 0+e],[0 1 1 1-e 1-e 0+e],c3);plot([0 1 1 0 0],[0 0 1 1 0]);
  wires:
  "p{1}"/1 -> Delays 1/1("p{1}")
  Delays 1/1("pd{1,1}") -> "IW{1,1}"/1("pd{1,1}")
  "IW{1,1}"/1("iz{1,1}") -> netsum/1
  "b{1}"/1 -> netsum/2
  netsum/1 -> tansig/1
  tansig/1 -> "a{1}"/1

== system dynamicANN/BEARING 1 NL1/B1NN/Layer 2 ==
  "a{1} " : Inport  PortDimensions=100
      mask Display: e = 0.06;c1 = [120 230 180]/255;c2 = ([120 230 180]+0)/(256+128);c3 = ([120 230 180]+128)/(256+128);patch([0 1 1 0],[0 0 1 1],c1);patch([0 1 1 1-e 1-e 0+e],[0 0 1 1-e 0+e 0+e],c2);patch([0 0 1 1-e 0+e 0+e],[0 1 1 1-e 1-e 0+e],c3);plot([0 1 1 0 0],[0 0 1 1 0]);
  Delays 1 : Subsystem
      mask Display: e = 0.06;c1 = [120 150 230]/255;c2 = ([120 150 230]+0)/383;c3 = ([120 150 230]+128)/383;patch([0 1 1 0],[0 0 1 1],c1);patch([0 1 1 1-e 1-e 0+e],[0 0 1 1-e 0+e 0+e],c2);patch([0 0 1 1-e 0+e 0+e],[0 1 1 1-e 1-e 0+e],c3);plot([0 1 1 0 0],[0 0 1 1 0]);disp('0');
  "LW{2,1}" : Subsystem
      mask Display: e = 0.06;c1 = [120 150 230]/255;c2 = ([120 150 230]+0)/383;c3 = ([120 150 230]+128)/383;patch([0 1 1 0],[0 0 1 1],c1);patch([0 1 1 1-e 1-e 0+e],[0 0 1 1-e 0+e 0+e],c2);patch([0 0 1 1-e 0+e 0+e],[0 1 1 1-e 1-e 0+e],c3);plot([0 1 1 0 0],[0 0 1 1 0]);disp('W');
  "b{2}" : Constant  Value=[0.324730286525802547270558306991006247699260711669921875;-0.321573246477363294815177141572348773479461669921875]
      mask Display: e = 0.06;c1 = [120 150 230]/255;c2 = ([120 150 230]+0)/383;c3 = ([120 150 230]+128)/383;patch([0 1 1 0],[0 0 1 1],c1);patch([0 1 1 1-e 1-e 0+e],[0 0 1 1-e 0+e 0+e],c2);patch([0 0 1 1-e 0+e 0+e],[0 1 1 1-e 1-e 0+e],c3);plot([0 1 1 0 0],[0 0 1 1 0]);disp('b');
  netsum : Sum  Inputs=2  SaturateOnIntegerOverflow=on  InputSameDT=on  OutDataTypeStr=Inherit: Same as first input
      mask Display: e = 0.06;c1 = [120 150 230]/255;c2 = ([120 150 230]+0)/383;c3 = ([120 150 230]+128)/383;patch([0 1 1 0],[0 0 1 1],c1);patch([0 1 1 1-e 1-e 0+e],[0 0 1 1-e 0+e 0+e],c2);patch([0 0 1 1-e 0+e 0+e],[0 1 1 1-e 1-e 0+e],c3);plot([0 1 1 0 0],[0 0 1 1 0]);disp('+');
  purelin : neural/Transfer Functions/purelin
      settings: SourceProductName=Deep Learning Toolbox
  "a{2}" : Outport  InitialOutput=[0;0]
      mask Display: e = 0.06;c1 = [120 230 180]/255;c2 = ([120 230 180]+0)/(256+128);c3 = ([120 230 180]+128)/(256+128);patch([0 1 1 0],[0 0 1 1],c1);patch([0 1 1 1-e 1-e 0+e],[0 0 1 1-e 0+e 0+e],c2);patch([0 0 1 1-e 0+e 0+e],[0 1 1 1-e 1-e 0+e],c3);plot([0 1 1 0 0],[0 0 1 1 0]);
  wires:
  "a{1} "/1 -> Delays 1/1("p{2}")
  Delays 1/1("pd{2,1}") -> "LW{2,1}"/1("ad{2,1}")
  "LW{2,1}"/1("lz{2,1}") -> netsum/1
  "b{2}"/1 -> netsum/2
  netsum/1 -> purelin/1
  purelin/1 -> "a{2}"/1

== system dynamicANN/BEARING 1 NL1/B1NN/Process Input 1 ==
  x : Inport  PortDimensions=4
      mask Display: e = 0.06;c1 = [120 230 180]/255;c2 = ([120 230 180]+0)/(256+128);c3 = ([120 230 180]+128)/(256+128);patch([0 1 1 0],[0 0 1 1],c1);patch([0 1 1 1-e 1-e 0+e],[0 0 1 1-e 0+e 0+e],c2);patch([0 0 1 1-e 0+e 0+e],[0 1 1 1-e 1-e 0+e],c3);plot([0 1 1 0 0],[0 0 1 1 0]);
  mapminmax : neural/Processing Functions/mapminmax  xmin=[-554.080025538255654282693285495;-135587.750697826064424589276314;-574.130831645498233228863682598;-163799.738536628108704462647438]  xmax=[490.857346777038515028834808618;123868.273609087846125476062298;503.884955189125548713491298258;98043.5266433354699984192848206]  ymin=-1  ymax=1
      settings: SourceProductName=Deep Learning Toolbox
  p : Outport  PortDimensions=4
      mask Display: e = 0.06;c1 = [120 230 180]/255;c2 = ([120 230 180]+0)/(256+128);c3 = ([120 230 180]+128)/(256+128);patch([0 1 1 0],[0 0 1 1],c1);patch([0 1 1 1-e 1-e 0+e],[0 0 1 1-e 0+e 0+e],c2);patch([0 0 1 1-e 0+e 0+e],[0 1 1 1-e 1-e 0+e],c3);plot([0 1 1 0 0],[0 0 1 1 0]);
  wires:
  x/1 -> mapminmax/1
  mapminmax/1 -> p/1

== system dynamicANN/BEARING 1 NL1/B1NN/Process Output 1 ==
  a : Inport  PortDimensions=2
      mask Display: e = 0.06;c1 = [120 230 180]/255;c2 = ([120 230 180]+0)/(256+128);c3 = ([120 230 180]+128)/(256+128);patch([0 1 1 0],[0 0 1 1],c1);patch([0 1 1 1-e 1-e 0+e],[0 0 1 1-e 0+e 0+e],c2);patch([0 0 1 1-e 0+e 0+e],[0 1 1 1-e 1-e 0+e],c3);plot([0 1 1 0 0],[0 0 1 1 0]);
  mapminmax_reverse : neural/Processing Functions/mapminmax_reverse  xmin=[-78.8835165544828527117715566419;-56.4640583704197354109055595472]  xmax=[81.9562261679372738853999180719;107.495790180707302852169959806]  ymin=-1  ymax=1
      settings: SourceProductName=Deep Learning Toolbox
  y : Outport  PortDimensions=2
      mask Display: e = 0.06;c1 = [120 230 180]/255;c2 = ([120 230 180]+0)/(256+128);c3 = ([120 230 180]+128)/(256+128);patch([0 1 1 0],[0 0 1 1],c1);patch([0 1 1 1-e 1-e 0+e],[0 0 1 1-e 0+e 0+e],c2);patch([0 0 1 1-e 0+e 0+e],[0 1 1 1-e 1-e 0+e],c3);plot([0 1 1 0 0],[0 0 1 1 0]);
  wires:
  a/1 -> mapminmax_reverse/1
  mapminmax_reverse/1 -> y/1

== system dynamicANN/BEARING 2 NL1/B2NN /Layer 1 ==
  "p{1}" : Inport  PortDimensions=4
      mask Display: e = 0.06;c1 = [120 230 180]/255;c2 = ([120 230 180]+0)/(256+128);c3 = ([120 230 180]+128)/(256+128);patch([0 1 1 0],[0 0 1 1],c1);patch([0 1 1 1-e 1-e 0+e],[0 0 1 1-e 0+e 0+e],c2);patch([0 0 1 1-e 0+e 0+e],[0 1 1 1-e 1-e 0+e],c3);plot([0 1 1 0 0],[0 0 1 1 0]);
  Delays 1 : Subsystem
      mask Display: e = 0.06;c1 = [120 150 230]/255;c2 = ([120 150 230]+0)/383;c3 = ([120 150 230]+128)/383;patch([0 1 1 0],[0 0 1 1],c1);patch([0 1 1 1-e 1-e 0+e],[0 0 1 1-e 0+e 0+e],c2);patch([0 0 1 1-e 0+e 0+e],[0 1 1 1-e 1-e 0+e],c3);plot([0 1 1 0 0],[0 0 1 1 0]);disp('0');
  "IW{1,1}" : Subsystem
      mask Display: e = 0.06;c1 = [120 150 230]/255;c2 = ([120 150 230]+0)/383;c3 = ([120 150 230]+128)/383;patch([0 1 1 0],[0 0 1 1],c1);patch([0 1 1 1-e 1-e 0+e],[0 0 1 1-e 0+e 0+e],c2);patch([0 0 1 1-e 0+e 0+e],[0 1 1 1-e 1-e 0+e],c3);plot([0 1 1 0 0],[0 0 1 1 0]);disp('W');
  "b{1}" : Constant  Value=[-0.2178309078748878191422733152649016119539737701416015625;-0.4663688232922715837247551462496630847454071044921875;1.0291205948709640782823271365487016737461090087890625;0.480309902987716530464723518889513798058032989501953125;1.161844801131203919197787399752996861934661865234375;-1.512967482361870619200772125623188912868499755859375;-0.273412838485520948150764297679415903985500335693359375;-0.94217390855659821635725847954745404422283172607421875;-0.07605758756975593282145808871064218692481517791748046875;-0.399790157521881794888685135447303764522075653076171875;0.79195210623637846136801954344264231622219085693359375;-3.192656660610529772981180940405465662479400634765625;-2.461688084332111170482448869734071195125579833984375;-0.1367343681641355335187881792080588638782501220703125;1.017505537075550581249672177364118397235870361328125;-2.093654754086606839535988910938613116741180419921875;0.9581022805738912406781082609086297452449798583984375;0.56402388946102177680330669318209402263164520263671875;0.71526576502755567776858924844418652355670928955078125;-0.91024327424186524115867769069154746830463409423828125;-0.70390847618132668106483151859720237553119659423828125;-4.40897960553333945199483423493802547454833984375;-2.973713982227526475554668650147505104541778564453125;1.0482416675917829440578543653828091919422149658203125;0.317549551932251372665660937855136580765247344970703125;0.731530098548386575885160709731280803680419921875;-2.675170120542511131844776173238642513751983642578125;1.8103766278381219212434416476753540337085723876953125;1.158265961724864734350148864905349910259246826171875;1.944688696809947714427835308015346527099609375;0.4034223551320514911111558831180445849895477294921875;0.0281655182581152345455688390529758180491626262664794921875;-0.150221987955851954410491089220158755779266357421875;-1.9341068217772769965989709817222319543361663818359375;-1.0238343643759808543336475850082933902740478515625;0.221748334588854678628422334440983831882476806640625;-0.9388198197484880491714420713833533227443695068359375;-2.0679451010865168569807792664505541324615478515625;-1.368368974507848445654190072673372924327850341796875;-2.735276600025368765045641339384019374847412109375;1.84503386751565212620107558905147016048431396484375;0.740345853366948691842708285548724234104156494140625;-0.5247589359035356171290231941384263336658477783203125;-1.56490918196444273036149752442725002765655517578125;0.63995198035091560573306423975736834108829498291015625;1.3379300699480338732172413074295036494731903076171875;-0.210387878801505279202643805547268129885196685791015625;2.797896808136826951596276558120734989643096923828125;-2.488271296185179171089885130641050636768341064453125;2.51543430575473525578900080290623009204864501953125;7.9013425365337486283578982693143188953399658203125;-0.470177644552810580780288773894426412880420684814453125;-2.0801539730077234224836502107791602611541748046875;2.062741497946209090486036075162701308727264404296875;-0.32071153368788285487056555211893282830715179443359375;-0.283212003982637627874652253012754954397678375244140625;1.0612309102350085954213909644749946892261505126953125;-1.1105087769466706060228489150176756083965301513671875;0.67348640024102934820149357619811780750751495361328125;0.10529861901466662510440386313348426483571529388427734375;0.391260940762822417848809664064901880919933319091796875;0.801509627119028511543774584424681961536407470703125;4.22541015087345517287076290813274681568145751953125;-1.4713116481372152666295960443676449358463287353515625;-0.283086075680045734515033473144285380840301513671875;1.2571731480514269918558056815527379512786865234375;-0.214181955816110713985978009077371098101139068603515625;-0.196712129894504650362563324961229227483272552490234375;-0.10797625994168437435494212195408181287348270416259765625;-6.52930735910772686025893563055433332920074462890625;-1.059147137326928334033482315135188400745391845703125;-2.74636677995498512672156721237115561962127685546875 ...(+1555 chars)]
      mask Display: e = 0.06;c1 = [120 150 230]/255;c2 = ([120 150 230]+0)/383;c3 = ([120 150 230]+128)/383;patch([0 1 1 0],[0 0 1 1],c1);patch([0 1 1 1-e 1-e 0+e],[0 0 1 1-e 0+e 0+e],c2);patch([0 0 1 1-e 0+e 0+e],[0 1 1 1-e 1-e 0+e],c3);plot([0 1 1 0 0],[0 0 1 1 0]);disp('b');
  netsum : Sum  Inputs=2  SaturateOnIntegerOverflow=on  InputSameDT=on  OutDataTypeStr=Inherit: Same as first input
      mask Display: e = 0.06;c1 = [120 150 230]/255;c2 = ([120 150 230]+0)/383;c3 = ([120 150 230]+128)/383;patch([0 1 1 0],[0 0 1 1],c1);patch([0 1 1 1-e 1-e 0+e],[0 0 1 1-e 0+e 0+e],c2);patch([0 0 1 1-e 0+e 0+e],[0 1 1 1-e 1-e 0+e],c3);plot([0 1 1 0 0],[0 0 1 1 0]);disp('+');
  tansig : neural/Transfer Functions/tansig
      settings: SourceProductName=Deep Learning Toolbox
  "a{1}" : Outport  InitialOutput=[0;0;0;0;0;0;0;0;0;0;0;0;0;0;0;0;0;0;0;0;0;0;0;0;0;0;0;0;0;0;0;0;0;0;0;0;0;0;0;0;0;0;0;0;0;0;0;0;0;0;0;0;0;0;0;0;0;0;0;0;0;0;0;0;0;0;0;0;0;0;0;0;0;0;0;0;0;0;0;0;0;0;0;0;0;0;0;0;0;0;0;0;0;0;0;0;0;0;0;0]
      mask Display: e = 0.06;c1 = [120 230 180]/255;c2 = ([120 230 180]+0)/(256+128);c3 = ([120 230 180]+128)/(256+128);patch([0 1 1 0],[0 0 1 1],c1);patch([0 1 1 1-e 1-e 0+e],[0 0 1 1-e 0+e 0+e],c2);patch([0 0 1 1-e 0+e 0+e],[0 1 1 1-e 1-e 0+e],c3);plot([0 1 1 0 0],[0 0 1 1 0]);
  wires:
  "p{1}"/1 -> Delays 1/1("p{1}")
  Delays 1/1("pd{1,1}") -> "IW{1,1}"/1("pd{1,1}")
  "IW{1,1}"/1("iz{1,1}") -> netsum/1
  "b{1}"/1 -> netsum/2
  netsum/1 -> tansig/1
  tansig/1 -> "a{1}"/1

== system dynamicANN/BEARING 2 NL1/B2NN /Layer 2 ==
  "a{1} " : Inport  PortDimensions=100
      mask Display: e = 0.06;c1 = [120 230 180]/255;c2 = ([120 230 180]+0)/(256+128);c3 = ([120 230 180]+128)/(256+128);patch([0 1 1 0],[0 0 1 1],c1);patch([0 1 1 1-e 1-e 0+e],[0 0 1 1-e 0+e 0+e],c2);patch([0 0 1 1-e 0+e 0+e],[0 1 1 1-e 1-e 0+e],c3);plot([0 1 1 0 0],[0 0 1 1 0]);
  Delays 1 : Subsystem
      mask Display: e = 0.06;c1 = [120 150 230]/255;c2 = ([120 150 230]+0)/383;c3 = ([120 150 230]+128)/383;patch([0 1 1 0],[0 0 1 1],c1);patch([0 1 1 1-e 1-e 0+e],[0 0 1 1-e 0+e 0+e],c2);patch([0 0 1 1-e 0+e 0+e],[0 1 1 1-e 1-e 0+e],c3);plot([0 1 1 0 0],[0 0 1 1 0]);disp('0');
  "LW{2,1}" : Subsystem
      mask Display: e = 0.06;c1 = [120 150 230]/255;c2 = ([120 150 230]+0)/383;c3 = ([120 150 230]+128)/383;patch([0 1 1 0],[0 0 1 1],c1);patch([0 1 1 1-e 1-e 0+e],[0 0 1 1-e 0+e 0+e],c2);patch([0 0 1 1-e 0+e 0+e],[0 1 1 1-e 1-e 0+e],c3);plot([0 1 1 0 0],[0 0 1 1 0]);disp('W');
  "b{2}" : Constant  Value=[-1.024314189728581681038122042082250118255615234375;1.068525411638810762582352253957651555538177490234375]
      mask Display: e = 0.06;c1 = [120 150 230]/255;c2 = ([120 150 230]+0)/383;c3 = ([120 150 230]+128)/383;patch([0 1 1 0],[0 0 1 1],c1);patch([0 1 1 1-e 1-e 0+e],[0 0 1 1-e 0+e 0+e],c2);patch([0 0 1 1-e 0+e 0+e],[0 1 1 1-e 1-e 0+e],c3);plot([0 1 1 0 0],[0 0 1 1 0]);disp('b');
  netsum : Sum  Inputs=2  SaturateOnIntegerOverflow=on  InputSameDT=on  OutDataTypeStr=Inherit: Same as first input
      mask Display: e = 0.06;c1 = [120 150 230]/255;c2 = ([120 150 230]+0)/383;c3 = ([120 150 230]+128)/383;patch([0 1 1 0],[0 0 1 1],c1);patch([0 1 1 1-e 1-e 0+e],[0 0 1 1-e 0+e 0+e],c2);patch([0 0 1 1-e 0+e 0+e],[0 1 1 1-e 1-e 0+e],c3);plot([0 1 1 0 0],[0 0 1 1 0]);disp('+');
  purelin : neural/Transfer Functions/purelin
      settings: SourceProductName=Deep Learning Toolbox
  "a{2}" : Outport  InitialOutput=[0;0]
      mask Display: e = 0.06;c1 = [120 230 180]/255;c2 = ([120 230 180]+0)/(256+128);c3 = ([120 230 180]+128)/(256+128);patch([0 1 1 0],[0 0 1 1],c1);patch([0 1 1 1-e 1-e 0+e],[0 0 1 1-e 0+e 0+e],c2);patch([0 0 1 1-e 0+e 0+e],[0 1 1 1-e 1-e 0+e],c3);plot([0 1 1 0 0],[0 0 1 1 0]);
  wires:
  "a{1} "/1 -> Delays 1/1("p{2}")
  Delays 1/1("pd{2,1}") -> "LW{2,1}"/1("ad{2,1}")
  "LW{2,1}"/1("lz{2,1}") -> netsum/1
  "b{2}"/1 -> netsum/2
  netsum/1 -> purelin/1
  purelin/1 -> "a{2}"/1
